simulink library "csc_imu_sensor_prep_mtv_lib"  (R2014b)
settings: Solver=ode45  SolverMode=SingleTasking  StartTime=0.0  StopTime=10.0  RelTol=1e-3
values from neighbouring files (symbols this model uses):
  kfl_use_mems = 1    [csc_kfl_kalman_filter_mtv_init.m]
  kfl_use_sensonor = 1    [csc_kfl_kalman_filter_mtv_init.m]
undefined symbols (not defined in the file or in its folder): mum1_dcm, sei_dcm, stg_body_to_head1_dcm, stg_miru_gyro_to_body_dcm
libraries: simulink x4, util_common_lib x4, util_event_lib x2, util_info_lib x1
settings Model: ExtModeAutoUpdateStatusClock=off  Creator=Administrator  LastModifiedBy=mstewart

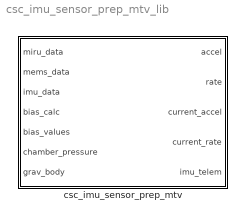
== system csc_imu_sensor_prep_mtv_lib ==
  csc_imu_sensor_prep_mtv : Subsystem

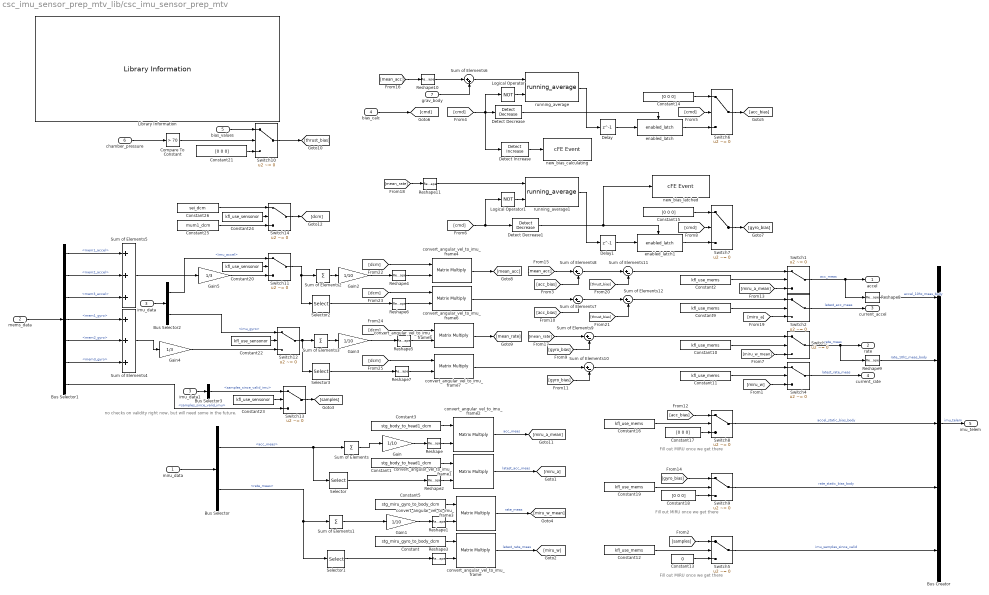
== system csc_imu_sensor_prep_mtv_lib/csc_imu_sensor_prep_mtv ==
  note: Fill out MIRU once we get there
  note: Fill out MIRU once we get there
  note: no checks on validity right now, but will need some in the future.
  note: Fill out MIRU once we get there
  miru_data : Inport
  mems_data : Inport  Port=2
  imu_data : Inport  Port=3
  bias_calc : Inport  Port=4
  bias_values : Inport  Port=5
  chamber_pressure : Inport  Port=6
  grav_body : Inport  Port=7
  Bus Creator : BusCreator  Inputs=5
  Bus Selector : BusSelector  OutputSignals=acc_meas,rate_meas
  Bus Selector1 : BusSelector  OutputSignals=mem1_accel,mem2_accel,mem3_accel,mem1_gyro,mem2_gyro,mem3_gyro,samples_since_valid_imu
  Bus Selector2 : BusSelector  OutputSignals=imu_accel,imu_gyro
  Bus Selector3 : BusSelector  OutputSignals=samples_since_valid_imu
  Compare To Constant : simulink/Logic and Bit Operations/Compare To Constant  relop=>  const=70  OutDataTypeStr=boolean
  Constant : Constant  Value=stg_miru_gyro_to_body_dcm
  Constant1 : Constant  Value=stg_body_to_head1_dcm
  Constant{2,9..12,16,19} (7 alike) : Constant  Value=kfl_use_mems
  Constant13 : Constant  Value=0  OutDataTypeStr=uint8
  Constant{14..15,17..18,21} (5 alike) : Constant  Value=[0 0 0]  OutDataTypeStr=double
  Constant{20,22..24} (4 alike) : Constant  Value=kfl_use_sensonor
  Constant25 : Constant  Value=mum1_dcm
  Constant26 : Constant  Value=sei_dcm
  Constant3 : Constant  Value=stg_body_to_head1_dcm
  Constant5 : Constant  Value=stg_miru_gyro_to_body_dcm
  Delay : Delay  DelayLength=1  InitialCondition=0
  Delay1 : Delay  DelayLength=1  InitialCondition=0
  Detect Decrease : simulink/Logic and Bit Operations/Detect Decrease  vinit=0.0  InputProcessing=Inherited  OutDataTypeStr=boolean
  Detect Decrease1 : simulink/Logic and Bit Operations/Detect Decrease  vinit=0.0  InputProcessing=Inherited  OutDataTypeStr=boolean
  Detect Increase : simulink/Logic and Bit Operations/Detect Increase  vinit=0.0  InputProcessing=Inherited  OutDataTypeStr=boolean
  Gain{,1..3} (4 alike) : Gain  Gain=1/10
  Gain4 : Gain  Gain=1/3
  Gain5 : Gain  Gain=1/3
  Library Information : util_info_lib/Library Information  owner='escrane'
  Logical Operator : Logic  Operator=NOT  AllPortsSameDT=off  OutDataTypeStr=boolean
  Logical Operator1 : Logic  Operator=NOT  AllPortsSameDT=off  OutDataTypeStr=boolean
  Reshape{,1..7} (8 alike) : Reshape  OutputDimensionality=Column vector (2-D)
  Reshape{8..11} (4 alike) : Reshape
  Selector{,1..3} (4 alike) : Selector  NumberOfDimensions=2  InputPortWidth=3  IndexOptions=Index vector (dialog),Select all  Indices=1,1  OutputSizes=1,1
  Sum of Elements{,1..3} (4 alike) : Sum  Inputs=+  CollapseMode=Specified dimension
  Sum of Elements{7..12} (6 alike) : Sum  Inputs=|+-  CollapseMode=Specified dimension
  Sum of Elements4 : Sum  Inputs=+++  CollapseMode=Specified dimension
  Sum of Elements5 : Sum  Inputs=+++  CollapseMode=Specified dimension
  Sum of Elements6 : Sum  Inputs=|++  CollapseMode=Specified dimension
  Switch{1..14} (14 alike) : Switch  Criteria=u2 ~= 0
  convert_angular_vel_to_imu_frame{,1..7} (8 alike) : Product  Multiplication=Matrix(*)  RndMeth=Zero
  enabled_latch : util_common_lib/enabled_latch  initial_output=0
  enabled_latch1 : util_common_lib/enabled_latch  initial_output=0
  imu_data1 : InportShadow  Port=3
  new_bias_calculating : util_event_lib/cFE Event  event_message='New IMU biases calculating'  event_id=67  event_severity=INFORMATION  event_use_enums=off  event_enum_types={}
  new_bias_latched : util_event_lib/cFE Event  event_message='New IMU biases latched'  event_id=68  event_severity=INFORMATION  event_use_enums=off  event_enum_types={}
  running_average : util_common_lib/running_average  initial_mean=[0 0 0]
  running_average1 : util_common_lib/running_average  initial_mean=[0 0 0]
  accel : Outport
  rate : Outport  Port=2
  current_accel : Outport  Port=3
  current_rate : Outport  Port=4
  imu_telem : Outport  Port=5
  wires:
  Switch14/1 -> [dcm]
  Constant26/1 -> Switch14/1
  Constant25/1 -> Switch14/3
  Constant24/1 -> Switch14/2
  Bus Selector3/1 -> Switch13/1  "<samples_since_valid_imu>"
  imu_data1/1 -> Bus Selector3/1
  Switch13/1 -> [samples]
  Constant23/1 -> Switch13/2
  Bus Selector2/2 -> Switch12/1  "<imu_gyro>"
  Gain4/1 -> Switch12/3
  Constant22/1 -> Switch12/2
  Bus Selector2/1 -> Switch11/1  "<imu_accel>"
  imu_data/1 -> Bus Selector2/1
  Gain5/1 -> Switch11/3
  Constant20/1 -> Switch11/2
  chamber_pressure/1 -> Compare To Constant/1
  Sum of Elements9/1 -> Switch3/1
  Sum of Elements11/1 -> Switch1/1
  Compare To Constant/1 -> Switch10/2
  Constant21/1 -> Switch10/3
  bias_values/1 -> Switch10/1
  Switch10/1 -> [thrust_bias]
  [thrust_bias] -> Sum of Elements12/2
  [thrust_bias] -> Sum of Elements11/2
  Sum of Elements12/1 -> Switch2/1
  Sum of Elements7/1 -> Sum of Elements12/1
  Sum of Elements8/1 -> Sum of Elements11/1
  Selector2/1 -> Reshape6/1
  [mean_rate] -> Sum of Elements9/1
  convert_angular_vel_to_imu_frame5/1 -> [mean_rate]
  [mean_acc] -> Sum of Elements8/1
  convert_angular_vel_to_imu_frame4/1 -> [mean_acc]
  Sum of Elements10/1 -> Switch4/1
  convert_angular_vel_to_imu_frame7/1 -> Sum of Elements10/1
  [mean_rate] -> Reshape11/1
  Gain3/1 -> Reshape5/1
  convert_angular_vel_to_imu_frame6/1 -> Sum of Elements7/1
  [mean_acc] -> Reshape10/1
  Gain2/1 -> Reshape4/1
  Selector3/1 -> Reshape7/1
  Bus Selector1/6 -> Sum of Elements4/3  "<mem3_gyro>"
  Bus Selector1/5 -> Sum of Elements4/2  "<mem2_gyro>"
  Reshape11/1 -> running_average1/1
  Reshape10/1 -> Sum of Elements6/1
  [gyro_bias] -> Sum of Elements10/2
  [gyro_bias] -> Sum of Elements9/2
  [acc_bias] -> Sum of Elements7/2
  [acc_bias] -> Sum of Elements8/2
  Detect Increase/1 -> new_bias_calculating/1
  Switch9/1 -> Bus Creator/4  "rate_static_bias_body"
  Constant18/1 -> Switch9/3
  Constant19/1 -> Switch9/2
  [gyro_bias] -> Switch9/1
  Switch8/1 -> Bus Creator/3  "accel_static_bias_body"
  Constant17/1 -> Switch8/3
  Constant16/1 -> Switch8/2
  [acc_bias] -> Switch8/1
  Constant15/1 -> Switch7/1
  [cmd] -> Switch7/2
  enabled_latch1/1 -> Switch7/3
  Switch7/1 -> [gyro_bias]
  Delay1/1 -> enabled_latch1/1
  Detect Decrease1/1 -> enabled_latch1/Enable, new_bias_latched/1
  Logical Operator1/1 -> running_average1/2
  running_average1/1 -> Delay1/1
  [cmd] -> Detect Decrease1/1, Logical Operator1/1
  Constant14/1 -> Switch6/1
  [cmd] -> Switch6/2
  grav_body/1 -> Sum of Elements6/2
  bias_calc/1 -> [cmd]
  enabled_latch/1 -> Switch6/3
  Switch6/1 -> [acc_bias]
  Delay/1 -> enabled_latch/1
  Sum of Elements6/1 -> running_average/1
  Detect Decrease/1 -> enabled_latch/Enable
  Logical Operator/1 -> running_average/2
  running_average/1 -> Delay/1
  [cmd] -> Detect Decrease/1, Logical Operator/1, Detect Increase/1
  Reshape9/1 -> Bus Creator/2  "rate_10hz_meas_body"
  Reshape8/1 -> Bus Creator/1  "accel_10hz_meas_body"
  Switch5/1 -> Bus Creator/5  "imu_samples_since_valid"
  Constant13/1 -> Switch5/3
  Constant12/1 -> Switch5/2
  [samples] -> Switch5/1
  Bus Selector1/7 -> Switch13/3  "<samples_since_valid_imu>"
  Bus Creator/1 -> imu_telem/1  "imu_telem"
  Switch4/1 -> current_rate/1  "latest_rate_meas"
  Switch3/1 -> rate/1, Reshape9/1  "rate_meas"
  [miru_w] -> Switch4/3
  [miru_w_mean] -> Switch3/3
  Constant11/1 -> Switch4/2
  Constant10/1 -> Switch3/2
  Switch2/1 -> current_accel/1  "latest_acc_meas"
  convert_angular_vel_to_imu_frame1/1 -> [miru_a]  "latest_acc_meas"
  [miru_a] -> Switch2/3
  [miru_a_mean] -> Switch1/3
  convert_angular_vel_to_imu_frame2/1 -> [miru_a_mean]  "acc_meas"
  Constant9/1 -> Switch2/2
  Switch1/1 -> accel/1, Reshape8/1  "acc_meas"
  Constant2/1 -> Switch1/2
  [dcm] -> convert_angular_vel_to_imu_frame7/1
  Reshape7/1 -> convert_angular_vel_to_imu_frame7/2
  [dcm] -> convert_angular_vel_to_imu_frame5/1
  [dcm] -> convert_angular_vel_to_imu_frame6/1
  Reshape6/1 -> convert_angular_vel_to_imu_frame6/2
  [dcm] -> convert_angular_vel_to_imu_frame4/1
  Sum of Elements4/1 -> Gain4/1
  Switch12/1 -> Sum of Elements3/1, Selector3/1
  Reshape5/1 -> convert_angular_vel_to_imu_frame5/2
  Sum of Elements3/1 -> Gain3/1
  Sum of Elements5/1 -> Gain5/1
  Switch11/1 -> Sum of Elements2/1, Selector2/1
  Bus Selector1/4 -> Sum of Elements4/1  "<mem1_gyro>"
  Reshape4/1 -> convert_angular_vel_to_imu_frame4/2
  Bus Selector1/3 -> Sum of Elements5/3  "<mem3_accel>"
  Bus Selector1/2 -> Sum of Elements5/2  "<mem2_accel>"
  Sum of Elements2/1 -> Gain2/1
  Bus Selector1/1 -> Sum of Elements5/1  "<mem1_accel>"
  mems_data/1 -> Bus Selector1/1
  Reshape3/1 -> convert_angular_vel_to_imu_frame/2
  Selector/1 -> Reshape2/1
  Reshape2/1 -> convert_angular_vel_to_imu_frame1/2
  Reshape1/1 -> convert_angular_vel_to_imu_frame3/2
  Reshape/1 -> convert_angular_vel_to_imu_frame2/2
  Sum of Elements1/1 -> Gain1/1
  Sum of Elements/1 -> Gain/1
  Constant5/1 -> convert_angular_vel_to_imu_frame3/1
  Gain1/1 -> Reshape1/1
  Bus Selector/2 -> Sum of Elements1/1, Selector1/1  "<rate_meas>"
  Gain/1 -> Reshape/1
  Constant3/1 -> convert_angular_vel_to_imu_frame2/1
  convert_angular_vel_to_imu_frame/1 -> [miru_w]  "latest_rate_meas"
  Selector1/1 -> Reshape3/1
  Constant1/1 -> convert_angular_vel_to_imu_frame1/1
  convert_angular_vel_to_imu_frame3/1 -> [miru_w_mean]  "rate_meas"
  Constant/1 -> convert_angular_vel_to_imu_frame/1
  Bus Selector/1 -> Sum of Elements/1, Selector/1  "<acc_meas>"
  miru_data/1 -> Bus Selector/1
